simulink model "sampleModel1617"  (R2023a)
settings: Solver=VariableStepAuto  StartTime=0.0  StopTime=10.0  RelTol=1e-3
libraries: hdlsllib x8, simulink x3
settings Model: Creator=user1  LastModifiedBy=user1

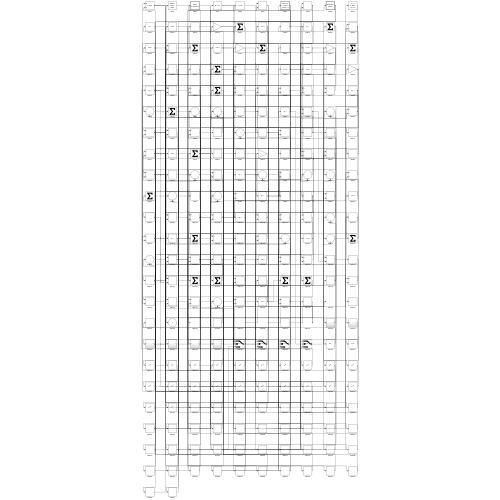
[thumbnail: Simulink's stored preview of the top-level diagram]
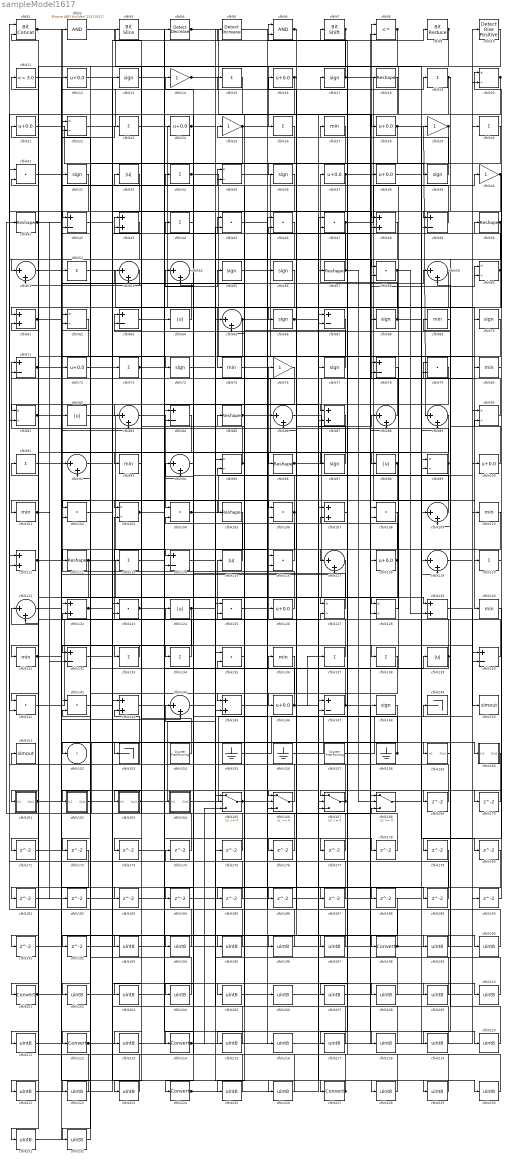
== system sampleModel1617 ==
  cfblk1 : hdlsllib/Logic and Bit Operations/Bit Concat  numInputs=2
  cfblk10 : hdlsllib/Logic and Bit Operations/Detect Rise Positive  vinit=0  OutDataTypeStr=boolean
  cfblk{12,16,21,24,28,37..38,72,100,118,126,146} (12 alike) : Bias  Bias=0.0  SaturateOnIntegerOverflow=off
  cfblk{27,69,75,80,93,101,110,130..131,136} (10 alike) : MinMax
  cfblk{31,45..47,58,79,102,104,106,108,116,123,125,135,141..142} (16 alike) : DotProduct  OutDataTypeStr=Inherit: Inherit via internal rule
  cfblk{20,22,35,60,62,81,90,95,99,103,127..128} (12 alike) : Product  Inputs=*/  RndMeth=Zero  SaturateOnIntegerOverflow=on
  cfblk{18,41,50,57,85,96,105,112} (8 alike) : Reshape
  cfblk{43,48,61,87,107,111,122,129,143,145} (10 alike) : Sum
  cfblk{51,53..54,59,65,83,86,88..89,92,94,109,117,119,121,144} (16 alike) : Sum  Inputs=|++
  cfblk11 : hdlsllib/Logic and Bit Operations/Compare To Constant  relop=<=  const=3.0  OutDataTypeStr=boolean
  cfblk{15,19,23,26,30,34,44,52,73,91,113,120,133..134,137..138} (16 alike) : Sum  Inputs=+
  cfblk{42,49,63,67,71,78,84,114,132,140,147} (11 alike) : Sum  Inputs=+-
  cfblk{33,64,82,98,115,124,139} (7 alike) : Abs  SaturateOnIntegerOverflow=off
  cfblk{13,17,32,36,39,55..56,66,68,70,74,77,97,148} (14 alike) : Signum
  cfblk{14,25,29,40,76} (5 alike) : Gain
  cfblk149 : Terminator
  cfblk150 : ToWorkspace  VariableName=simout  SaveFormat=Timeseries  SampleTime=-1
  cfblk151 : ToWorkspace  VariableName=simout  SaveFormat=Timeseries  SampleTime=-1
  cfblk153 : Terminator
  cfblk154 : hdlsllib/Sources/Counter Free-Running  NumBits=16  tsamp=-1
  cfblk155 : Ground
  cfblk156 : Ground
  cfblk157 : hdlsllib/Sources/Counter Free-Running  NumBits=16  tsamp=-1
  cfblk158 : Ground
  cfblk159 : Subsystem
      settings: LibrarySourceBlock=|
      | hdlsllib/Ports &
      | Subsystems/Subsystem
  cfblk160 : Subsystem
      settings: LibrarySourceBlock=|
      | hdlsllib/Ports &
      | Subsystems/Subsystem
  cfblk161 : Subsystem
      settings: LibrarySourceBlock=|
      | hdlsllib/Ports &
      | Subsystems/Subsystem
  cfblk162 : Subsystem
      settings: LibrarySourceBlock=|
      | hdlsllib/Ports &
      | Subsystems/Subsystem
  cfblk163 : Subsystem
      settings: LibrarySourceBlock=|
      | hdlsllib/Ports &
      | Subsystems/Subsystem
  cfblk164 : Subsystem
      settings: LibrarySourceBlock=|
      | hdlsllib/Ports &
      | Subsystems/Subsystem
  cfblk{165..168} (4 alike) : Switch  SaturateOnIntegerOverflow=off  InputSameDT=off
  cfblk{169..192} (24 alike) : Delay  SampleTime=1
  cfblk{193..197,199..200,202..211,213,215..223,225..226,228..232} (34 alike) : DataTypeConversion  OutDataTypeStr=uint8  SaturateOnIntegerOverflow=off  RndMeth=Floor
  cfblk{198,201,212,214,224,227} (6 alike) : DataTypeConversion  SaturateOnIntegerOverflow=off  RndMeth=Floor
  cfblk2 : simulink/Logic and Bit Operations/Bitwise Operator  logicop=AND  UseBitMask=on  BitMask=bin2dec('11011001')  BitMaskRealWorld=Stored Integer
      settings: LibrarySourceBlock=|
      | hdlsllib/Logic and Bit
      | Operations/Bitwise
      | Operator
  cfblk3 : hdlsllib/Logic and Bit Operations/Bit Slice  lidx=7  ridx=0
  cfblk4 : simulink/Logic and Bit Operations/Detect Decrease  vinit=0.0  OutDataTypeStr=boolean
      settings: LibrarySourceBlock=|
      | hdlsllib/Logic and Bit
      | Operations/Detect
      | Decrease
  cfblk5 : simulink/Logic and Bit Operations/Detect Increase  vinit=0.0  OutDataTypeStr=boolean
      settings: LibrarySourceBlock=|
      | hdlsllib/Logic and Bit
      | Operations/Detect
      | Increase
  cfblk6 : Logic  AllPortsSameDT=off  OutDataTypeStr=boolean
  cfblk7 : hdlsllib/Logic and Bit Operations/Bit Shift  mode=Shift Left Logical  N=0
  cfblk8 : RelationalOperator  Operator=<=  OutDataTypeStr=boolean  InputSameDT=off
  cfblk9 : hdlsllib/Logic and Bit Operations/Bit Reduce  mode=AND
  cfblk152 : Outport  VectorParamsAs1DForOutWhenUnconnected=off
  wires:
  cfblk126/1 -> cfblk2/1
  cfblk78/1 -> cfblk136/1
  cfblk109/1 -> cfblk82/1
  cfblk35/1 -> cfblk130/1
  cfblk6/1 -> cfblk106/1, cfblk196/1
  cfblk26/1 -> cfblk162/1(In1)
  cfblk56/1 -> cfblk75/1
  cfblk82/1 -> cfblk114/1
  cfblk9/1 -> cfblk112/1, cfblk28/1
  cfblk100/1 -> cfblk63/1
  cfblk43/1 -> cfblk111/2
  cfblk30/1 -> cfblk83/1
  cfblk39/1 -> cfblk25/1
  cfblk23/1 -> cfblk66/1
  cfblk86/1 -> cfblk128/1
  cfblk99/1 -> cfblk71/1, cfblk146/1
  cfblk76/1 -> cfblk131/1
  cfblk148/1 -> cfblk41/1
  cfblk59/1 -> cfblk103/1
  cfblk117/1 -> cfblk161/1(In1)
  cfblk28/1 -> cfblk89/1, cfblk152/1
  cfblk98/1 -> cfblk163/1(In1), cfblk105/1
  cfblk65/1 -> cfblk101/1, cfblk48/2
  cfblk66/1 -> cfblk209/1, cfblk228/1
  cfblk47/1 -> cfblk40/1, cfblk223/1
  cfblk123/1 -> cfblk178/1, cfblk218/1
  cfblk50/1 -> cfblk169/1, cfblk232/1
  cfblk167/1 -> cfblk151/1, cfblk143/2
  cfblk127/1 -> cfblk34/1
  cfblk88/1 -> cfblk8/1
  cfblk120/1 -> cfblk50/1
  cfblk137/1 -> cfblk76/1
  cfblk49/1 -> cfblk32/1
  cfblk8/1 -> cfblk51/1, cfblk117/1
  cfblk17/1 -> cfblk120/1, cfblk6/1
  cfblk143/1 -> cfblk139/1
  cfblk1/1 -> cfblk74/1, cfblk99/2, cfblk106/2
  cfblk68/1 -> cfblk37/1, cfblk60/1
  cfblk134/1 -> cfblk103/2
  cfblk54/1 -> cfblk224/1
  cfblk44/1 -> cfblk214/1
  cfblk55/1 -> cfblk80/1
  cfblk61/1 -> cfblk122/1, cfblk33/1, cfblk83/2
  cfblk70/1 -> cfblk102/1
  cfblk18/1 -> cfblk42/1
  cfblk32/1 -> cfblk61/1
  cfblk90/1 -> cfblk17/1
  cfblk128/1 -> cfblk38/1
  cfblk24/1 -> cfblk116/2, cfblk197/1
  cfblk161/1(Out1) -> cfblk59/1, cfblk187/1
  cfblk4/1 -> cfblk68/1, cfblk208/1
  cfblk3/1 -> cfblk64/1
  cfblk31/1 -> cfblk198/1
  cfblk141/1 -> cfblk115/1
  cfblk52/1 -> cfblk119/1
  cfblk51/1 -> cfblk12/1
  cfblk95/1 -> cfblk43/1, cfblk215/1
  cfblk158/1 -> cfblk85/1, cfblk122/2
  cfblk85/1 -> cfblk10/1, cfblk97/1
  cfblk37/1 -> cfblk39/1, cfblk141/2, cfblk88/2
  cfblk53/1 -> cfblk51/2
  cfblk19/1 -> cfblk49/1, cfblk58/2
  cfblk63/1 -> cfblk98/1
  cfblk48/1 -> cfblk128/2
  cfblk57/1 -> cfblk27/1, cfblk16/1, cfblk168/2
  cfblk166/1 -> cfblk124/1
  cfblk16/1 -> cfblk145/1, cfblk86/2, cfblk194/1
  cfblk14/1 -> cfblk77/1, cfblk189/1
  cfblk10/1 -> cfblk26/1
  cfblk96/1 -> cfblk29/1, cfblk60/2
  cfblk156/1 -> cfblk149/1
  cfblk58/1 -> cfblk81/1, cfblk129/2
  cfblk119/1 -> cfblk30/1
  cfblk132/1 -> cfblk13/1
  cfblk64/1 -> cfblk52/1
  cfblk135/1 -> cfblk35/1
  cfblk2/1 -> cfblk119/2
  cfblk121/1 -> cfblk227/1
  cfblk83/1 -> cfblk104/1
  cfblk77/1 -> cfblk53/1
  cfblk146/1 -> cfblk88/1, cfblk63/2, cfblk137/1, cfblk22/2
  cfblk102/1 -> cfblk167/2
  cfblk122/1 -> cfblk160/1(In1), cfblk9/1
  cfblk116/1 -> cfblk104/2
  cfblk73/1 -> cfblk5/1, cfblk167/3, cfblk87/2
  cfblk140/1 -> cfblk7/1
  cfblk154/1 -> cfblk53/2
  cfblk40/1 -> cfblk70/1, cfblk113/1
  cfblk163/1(Out1) -> cfblk3/1, cfblk45/2
  cfblk106/1 -> cfblk95/2, cfblk173/1
  cfblk25/1 -> cfblk145/2, cfblk67/2
  cfblk165/1 -> cfblk126/1, cfblk168/3
  cfblk29/1 -> cfblk87/1, cfblk165/2
  cfblk34/1 -> cfblk118/1, cfblk58/1
  cfblk81/1 -> cfblk93/1, cfblk166/2, cfblk183/1
  cfblk27/1 -> cfblk96/1
  cfblk80/1 -> cfblk20/1
  cfblk87/1 -> cfblk114/2
  cfblk84/1 -> cfblk201/1
  cfblk133/1 -> cfblk132/1
  cfblk157/1 -> cfblk109/1
  cfblk139/1 -> cfblk91/1, cfblk109/2, cfblk135/2
  cfblk118/1 -> cfblk147/2, cfblk65/2
  cfblk21/1 -> cfblk78/1
  cfblk97/1 -> cfblk71/2
  cfblk104/1 -> cfblk20/2, cfblk79/2
  cfblk168/1 -> cfblk99/1
  cfblk41/1 -> cfblk117/2, cfblk132/2, cfblk15/1, cfblk191/1
  cfblk91/1 -> cfblk19/1
  cfblk74/1 -> cfblk140/2
  cfblk159/1(Out1) -> cfblk59/2
  cfblk15/1 -> cfblk81/2
  cfblk105/1 -> cfblk133/1
  cfblk60/1 -> cfblk14/1, cfblk166/3
  cfblk131/1 -> cfblk35/2, cfblk127/2
  cfblk7/1 -> cfblk141/1, cfblk203/1
  cfblk111/1 -> cfblk144/2, cfblk23/1
  cfblk147/1 -> cfblk86/1, cfblk220/1
  cfblk113/1 -> cfblk166/1
  cfblk71/1 -> cfblk159/1(In1), cfblk127/1, cfblk138/1
  cfblk5/1 -> cfblk56/1
  cfblk112/1 -> cfblk129/1, cfblk6/2, cfblk171/1
  cfblk129/1 -> cfblk150/1
  cfblk67/1 -> cfblk134/1
  cfblk103/1 -> cfblk55/1, cfblk177/1
  cfblk20/1 -> cfblk36/1, cfblk78/2
  cfblk42/1 -> cfblk48/1
  cfblk164/1(Out1) -> cfblk116/1
  cfblk155/1 -> cfblk100/1
  cfblk124/1 -> cfblk79/1, cfblk222/1
  cfblk22/1 -> cfblk4/1
  cfblk162/1(Out1) -> cfblk45/1
  cfblk36/1 -> cfblk153/1
  cfblk115/1 -> cfblk94/1
  cfblk110/1 -> cfblk212/1
  cfblk101/1 -> cfblk181/1, cfblk182/1
  cfblk169/1 -> cfblk1/1
  cfblk160/1(Out1) -> cfblk170/1
  cfblk170/1 -> cfblk167/1
  cfblk171/1 -> cfblk102/2
  cfblk136/1 -> cfblk172/1
  cfblk174/1 -> cfblk43/2
  cfblk114/1 -> cfblk175/1
  cfblk175/1 -> cfblk144/1
  cfblk79/1 -> cfblk176/1
  cfblk176/1 -> cfblk1/2
  cfblk177/1 -> cfblk143/1
  cfblk178/1 -> cfblk147/1
  cfblk130/1 -> cfblk179/1
  cfblk38/1 -> cfblk180/1
  cfblk181/1 -> cfblk165/1
  cfblk182/1 -> cfblk65/1
  cfblk183/1 -> cfblk95/1
  cfblk94/1 -> cfblk184/1
  cfblk184/1 -> cfblk49/2
  cfblk138/1 -> cfblk185/1
  cfblk185/1 -> cfblk111/1
  cfblk12/1 -> cfblk186/1
  cfblk186/1 -> cfblk8/2
  cfblk187/1 -> cfblk142/1
  cfblk45/1 -> cfblk188/1
  cfblk189/1 -> cfblk22/1
  cfblk190/1 -> cfblk90/2
  cfblk191/1 -> cfblk47/1
  cfblk33/1 -> cfblk192/1
  cfblk192/1 -> cfblk140/1
  cfblk11/1 -> cfblk193/1
  cfblk193/1 -> cfblk24/1
  cfblk194/1 -> cfblk11/1
  cfblk46/1 -> cfblk195/1
  cfblk195/1 -> cfblk21/1
  cfblk196/1 -> cfblk46/1
  cfblk197/1 -> cfblk46/2
  cfblk198/1 -> cfblk61/2, cfblk90/1
  cfblk75/1 -> cfblk199/1
  cfblk199/1 -> cfblk31/1
  cfblk173/1 -> cfblk200/1
  cfblk200/1 -> cfblk31/2
  cfblk201/1 -> cfblk164/1(In1), cfblk73/1
  cfblk188/1 -> cfblk202/1
  cfblk202/1 -> cfblk84/1
  cfblk203/1 -> cfblk84/2
  cfblk108/1 -> cfblk204/1
  cfblk204/1 -> cfblk42/2
  cfblk13/1 -> cfblk205/1
  cfblk205/1 -> cfblk108/1
  cfblk145/1 -> cfblk206/1
  cfblk206/1 -> cfblk108/2
  cfblk107/1 -> cfblk207/1
  cfblk207/1 -> cfblk190/1
  cfblk208/1 -> cfblk107/1
  cfblk209/1 -> cfblk107/2
  cfblk72/1 -> cfblk210/1
  cfblk210/1 -> cfblk135/1
  cfblk89/1 -> cfblk211/1
  cfblk211/1 -> cfblk72/1
  cfblk212/1 -> cfblk94/2, cfblk18/1
  cfblk93/1 -> cfblk213/1
  cfblk213/1 -> cfblk110/1
  cfblk214/1 -> cfblk168/1, cfblk165/3, cfblk148/1
  cfblk215/1 -> cfblk44/1
  cfblk125/1 -> cfblk216/1
  cfblk216/1 -> cfblk89/2
  cfblk179/1 -> cfblk217/1
  cfblk217/1 -> cfblk125/1
  cfblk218/1 -> cfblk125/2
  cfblk69/1 -> cfblk219/1
  cfblk219/1 -> cfblk123/1
  cfblk220/1 -> cfblk69/1
  cfblk62/1 -> cfblk221/1
  cfblk221/1 -> cfblk123/2
  cfblk222/1 -> cfblk62/1
  cfblk223/1 -> cfblk62/2
  cfblk224/1 -> cfblk67/1, cfblk57/1
  cfblk180/1 -> cfblk225/1
  cfblk225/1 -> cfblk54/1
  cfblk142/1 -> cfblk226/1
  cfblk226/1 -> cfblk54/2
  cfblk227/1 -> cfblk174/1, cfblk142/2
  cfblk228/1 -> cfblk121/1
  cfblk144/1 -> cfblk229/1
  cfblk229/1 -> cfblk121/2
  cfblk92/1 -> cfblk230/1
  cfblk230/1 -> cfblk47/2
  cfblk172/1 -> cfblk231/1
  cfblk231/1 -> cfblk92/1
  cfblk232/1 -> cfblk92/2

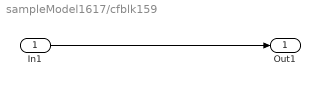
== system sampleModel1617/cfblk159 ==
  In1 : Inport
  Out1 : Outport
  wires:
  In1/1 -> Out1/1

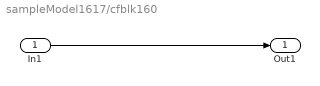
== system sampleModel1617/cfblk160 ==
  In1 : Inport
  Out1 : Outport
  wires:
  In1/1 -> Out1/1

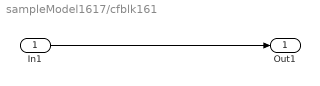
== system sampleModel1617/cfblk161 ==
  In1 : Inport
  Out1 : Outport
  wires:
  In1/1 -> Out1/1

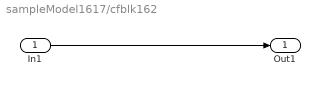
== system sampleModel1617/cfblk162 ==
  In1 : Inport
  Out1 : Outport
  wires:
  In1/1 -> Out1/1

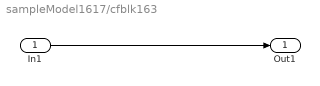
== system sampleModel1617/cfblk163 ==
  In1 : Inport
  Out1 : Outport
  wires:
  In1/1 -> Out1/1

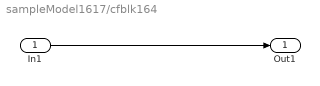
== system sampleModel1617/cfblk164 ==
  In1 : Inport
  Out1 : Outport
  wires:
  In1/1 -> Out1/1
